simulink model "cic"  (Simulink 6.3)
settings: Solver=FixedStepDiscrete  SolverMode=SingleTasking  StartTime=0.0  StopTime=1000  RelTol=1e-3
InitFcn:
  | %% DSPBuilder Start
  | alt_dspbuilder_update_model(bdroot)
  | %% DSPBuilder End
libraries: allblocks_alteradspbuilder2 x32
settings Model: Creator=mjervis  LastModifiedBy=LKONG
settings DataIOCC: SignalLoggingName=sigsOut
settings OptimizationCC: BooleanDataType=off  InlineInvariantSignals=on
settings DebuggingCC: SolverPrmCheckMsg=none
settings HardwareCC: TargetUnknown=on

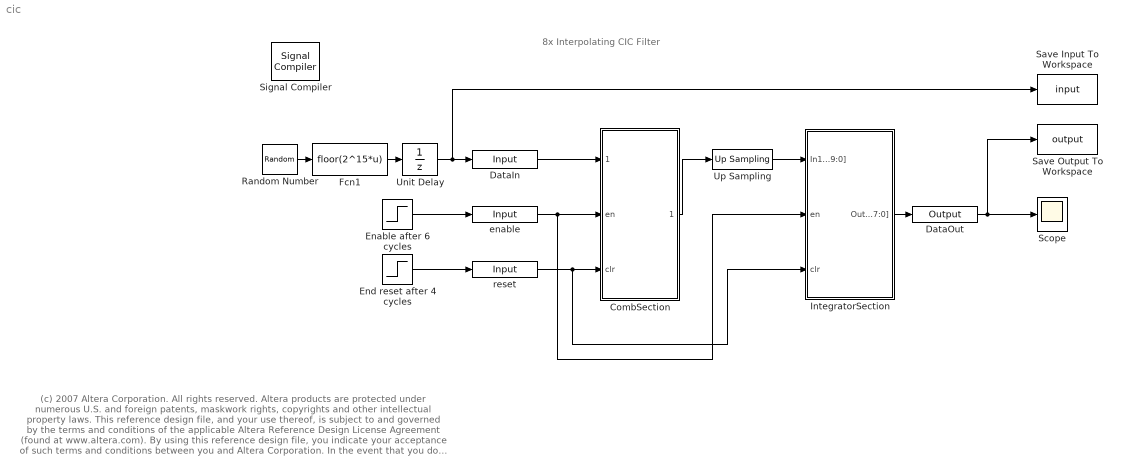
== system cic ==
  note: 8x Interpolating CIC Filter
  note: (c) 2007 Altera Corporation. All rights reserved.  Altera products are protected under numerous U.S. and foreign patents, maskwork rights, copyrights and other intellectual property laws.
      | This reference design file, and your use thereof, is subject to and governed by the terms and conditions of the applicable Altera Reference Design License Agreement (found at www.altera.com).
      | By using this reference design file, you indicate your acceptance of such terms and conditions between you and Altera Corporation.
      | In the event that you do not agree with such terms and conditions, you may not use the reference design file and please promptly destroy any copies you have made.
      | This reference design file being provided on an "as-is" basis and as an accommodation and therefore all warranties, representations or guarantees of any kind (whether express, implied or statutory)
      | including, without limitation, warranties of merchantability, non-infringement, or fitness for a particular purpose, are specifically disclaimed.
      | By making this reference design file available, Altera expressly does not recommend, suggest or require that this reference design file be used in combination with any other product not provided by Altera
  CombSection : Subsystem  AncestorBlock=ALTELINK/AltLab/HDL SubSystem
      mask Type: SubSystem AlteraBlockSet
  DataIn : allblocks_alteradspbuilder2/Input  iofile=D:\wsTrunk\workspace\Documentation\DesignExamples\Demos\Filters\CicFilter\Cic\tb_cic\cic_DataIn.salt  BusType=Signed Integer  bwl=16  bwr=0  SpecifyClock=off  PORTTYPE=Input
  DataOut : allblocks_alteradspbuilder2/Output  iofile=D:\wsTrunk\workspace\Documentation\DesignExamples\Demos\Filters\CicFilter\Cic\tb_cic\cic_DataOut.capture  BusType=Signed Integer  bwl=28  bwr=0  PORTTYPE=Output
  Enable after 6 cycles : Step  Time=6  SampleTime=1
  End reset after 4 cycles : Step  Time=4  Before=1  After=0  SampleTime=1
  Fcn1 : Fcn  Expr=floor(2^15*u)
  IntegratorSection : Subsystem  AncestorBlock=ALTELINK/AltLab/HDL SubSystem
      mask Type: SubSystem AlteraBlockSet
  Random Number : RandomNumber  Variance=8  SampleTime=8
  Save Input To Workspace : ToWorkspace  VariableName=input  SampleTime=-1  SaveFormat=Array
  Save Output To Workspace : ToWorkspace  VariableName=output  SampleTime=-1  SaveFormat=Array
  Scope : Scope
      settings: TimeRange=1000  YMin=-150000000  YMax=150000000  SaveName=ScopeData2
  Signal Compiler : allblocks_alteradspbuilder2/Signal Compiler  DeviceFamily=Stratix IV  DeviceName=AUTO  EnableSignalTap=off  SignalTapDepth=128  UseBoardBlock=off  StpUseDefaultClock=on  StpClock=Clock
  Unit Delay : UnitDelay  SampleTime=8
  Up Sampling : allblocks_alteradspbuilder2/Up Sampling  rate=8
  enable : allblocks_alteradspbuilder2/Input  iofile=D:\wsTrunk\workspace\Documentation\DesignExamples\Demos\Filters\CicFilter\Cic\tb_cic\cic_enable.salt  BusType=Single Bit  bwl=1  bwr=0  SpecifyClock=off  PORTTYPE=Input
  reset : allblocks_alteradspbuilder2/Input  iofile=D:\wsTrunk\workspace\Documentation\DesignExamples\Demos\Filters\CicFilter\Cic\tb_cic\cic_reset.salt  BusType=Single Bit  bwl=1  bwr=0  SpecifyClock=off  PORTTYPE=Input
  wires:
  Up Sampling/1 -> IntegratorSection/1(In1[19:0])
  IntegratorSection/1(Out1[27:0]) -> DataOut/1
  DataOut/1 -> Scope/1, Save Output To Workspace/1
  Random Number/1 -> Fcn1/1
  Unit Delay/1 -> DataIn/1, Save Input To Workspace/1
  Fcn1/1 -> Unit Delay/1
  CombSection/1(Out1[20:0]) -> Up Sampling/1
  Enable after 6 cycles/1 -> enable/1
  End reset after 4 cycles/1 -> reset/1
  DataIn/1 -> CombSection/1(In1[16:0])
  enable/1 -> CombSection/2(en), IntegratorSection/2(en)
  reset/1 -> IntegratorSection/3(clr), CombSection/3(clr)

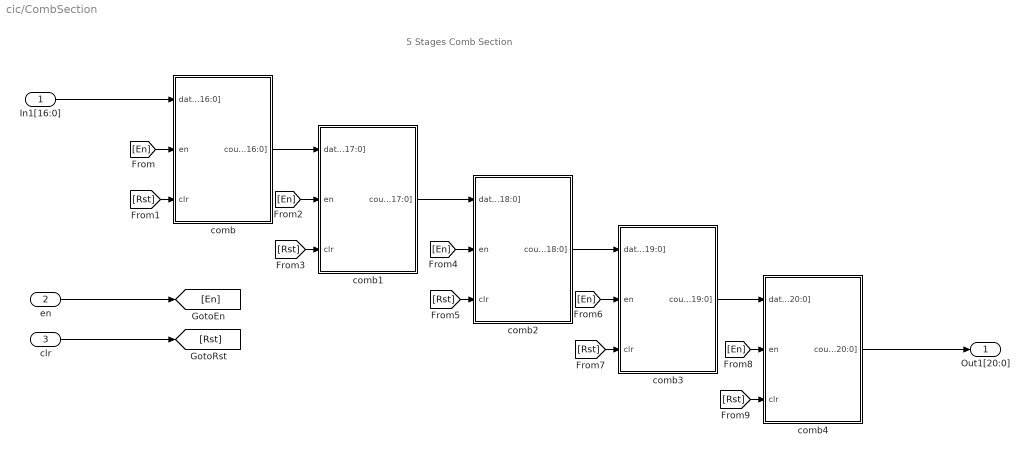
== system cic/CombSection ==
  note: 5 Stages Comb Section
  In1[16:0] : Inport
  en : Inport  Port=2
  clr : Inport  Port=3
  comb : Subsystem  AncestorBlock=ALTELINK/AltLab/HDL SubSystem
      mask Type: SubSystem AlteraBlockSet
  comb1 : Subsystem  AncestorBlock=ALTELINK/AltLab/HDL SubSystem
      mask Type: SubSystem AlteraBlockSet
  comb2 : Subsystem  AncestorBlock=ALTELINK/AltLab/HDL SubSystem
      mask Type: SubSystem AlteraBlockSet
  comb3 : Subsystem  AncestorBlock=ALTELINK/AltLab/HDL SubSystem
      mask Type: SubSystem AlteraBlockSet
  comb4 : Subsystem  AncestorBlock=ALTELINK/AltLab/HDL SubSystem
      mask Type: SubSystem AlteraBlockSet
  Out1[20:0] : Outport
  wires:
  In1[16:0]/1 -> comb/1(data[16:0])
  comb/1(cout[16:0]) -> comb1/1(data[17:0])
  comb1/1(cout[17:0]) -> comb2/1(data[18:0])
  comb2/1(cout[18:0]) -> comb3/1(data[19:0])
  comb3/1(cout[19:0]) -> comb4/1(data[20:0])
  comb4/1(cout[20:0]) -> Out1[20:0]/1
  en/1 -> [En]
  clr/1 -> [Rst]
  [En] -> comb/2(en)
  [Rst] -> comb/3(clr)
  [En] -> comb4/2(en)
  [Rst] -> comb4/3(clr)
  [En] -> comb3/2(en)
  [Rst] -> comb3/3(clr)
  [En] -> comb2/2(en)
  [Rst] -> comb2/3(clr)
  [En] -> comb1/2(en)
  [Rst] -> comb1/3(clr)

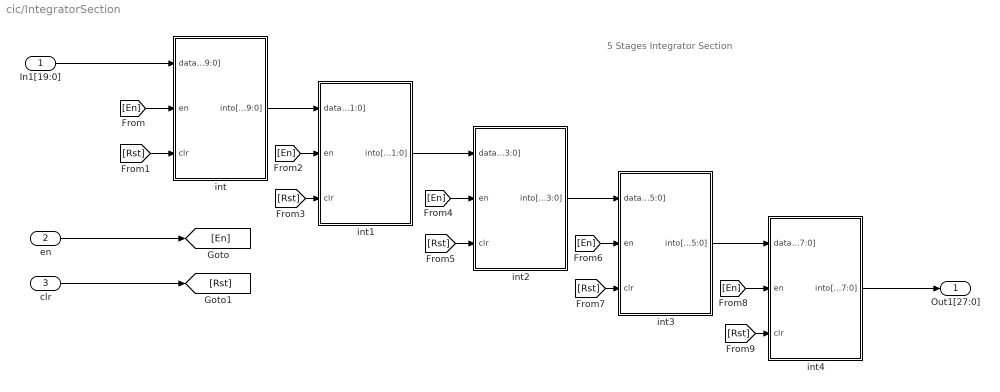
== system cic/IntegratorSection ==
  note: 5 Stages Integrator Section
  In1[19:0] : Inport
  en : Inport  Port=2
  clr : Inport  Port=3
  int : Subsystem  AncestorBlock=ALTELINK/AltLab/HDL SubSystem
      mask Type: SubSystem AlteraBlockSet
  int1 : Subsystem  AncestorBlock=ALTELINK/AltLab/HDL SubSystem
      mask Type: SubSystem AlteraBlockSet
  int2 : Subsystem  AncestorBlock=ALTELINK/AltLab/HDL SubSystem
      mask Type: SubSystem AlteraBlockSet
  int3 : Subsystem  AncestorBlock=ALTELINK/AltLab/HDL SubSystem
      mask Type: SubSystem AlteraBlockSet
  int4 : Subsystem  AncestorBlock=ALTELINK/AltLab/HDL SubSystem
      mask Type: SubSystem AlteraBlockSet
  Out1[27:0] : Outport
  wires:
  In1[19:0]/1 -> int/1(data[19:0])
  int/1(into[19:0]) -> int1/1(data[21:0])
  int1/1(into[21:0]) -> int2/1(data[23:0])
  int2/1(into[23:0]) -> int3/1(data[25:0])
  int3/1(into[25:0]) -> int4/1(data[27:0])
  en/1 -> [En]
  clr/1 -> [Rst]
  int4/1(into[27:0]) -> Out1[27:0]/1
  [En] -> int/2(en)
  [Rst] -> int/3(clr)
  [En] -> int4/2(en)
  [Rst] -> int4/3(clr)
  [En] -> int3/2(en)
  [Rst] -> int3/3(clr)
  [En] -> int2/2(en)
  [Rst] -> int2/3(clr)
  [En] -> int1/2(en)
  [Rst] -> int1/3(clr)

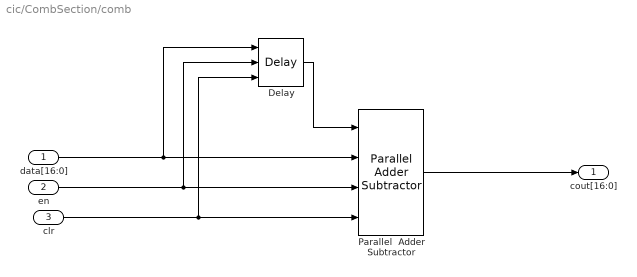
== system cic/CombSection/comb ==
  data[16:0] : Inport
  en : Inport  Port=2
  clr : Inport  Port=3
  Delay : allblocks_alteradspbuilder2/Delay  pipeline=1  ClockPhase=10000000  use_ena=on  use_sclr=on  use_init=off  reset_value=1
  Parallel  Adder Subtractor : allblocks_alteradspbuilder2/Parallel Adder Subtractor  number_of_inputs=2  direction=-  use_pipeline=on  phase_selection=10000000  use_ena=on  use_aclr=on
  cout[16:0] : Outport
  wires:
  Delay/1 -> Parallel  Adder Subtractor/1
  Parallel  Adder Subtractor/1 -> cout[16:0]/1
  en/1 -> Parallel  Adder Subtractor/3, Delay/2
  clr/1 -> Parallel  Adder Subtractor/4, Delay/3
  data[16:0]/1 -> Parallel  Adder Subtractor/2, Delay/1

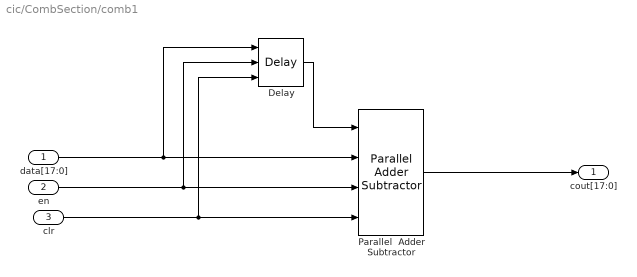
== system cic/CombSection/comb1 ==
  data[17:0] : Inport
  en : Inport  Port=2
  clr : Inport  Port=3
  Delay : allblocks_alteradspbuilder2/Delay  pipeline=1  ClockPhase=10000000  use_ena=on  use_sclr=on  use_init=off  reset_value=1
  Parallel  Adder Subtractor : allblocks_alteradspbuilder2/Parallel Adder Subtractor  number_of_inputs=2  direction=-  use_pipeline=on  phase_selection=10000000  use_ena=on  use_aclr=on
  cout[17:0] : Outport
  wires:
  Delay/1 -> Parallel  Adder Subtractor/1
  Parallel  Adder Subtractor/1 -> cout[17:0]/1
  en/1 -> Parallel  Adder Subtractor/3, Delay/2
  clr/1 -> Parallel  Adder Subtractor/4, Delay/3
  data[17:0]/1 -> Parallel  Adder Subtractor/2, Delay/1

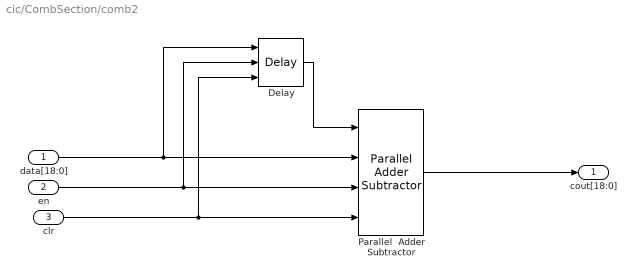
== system cic/CombSection/comb2 ==
  data[18:0] : Inport
  en : Inport  Port=2
  clr : Inport  Port=3
  Delay : allblocks_alteradspbuilder2/Delay  pipeline=1  ClockPhase=10000000  use_ena=on  use_sclr=on  use_init=off  reset_value=1
  Parallel  Adder Subtractor : allblocks_alteradspbuilder2/Parallel Adder Subtractor  number_of_inputs=2  direction=-  use_pipeline=on  phase_selection=10000000  use_ena=on  use_aclr=on
  cout[18:0] : Outport
  wires:
  data[18:0]/1 -> Delay/1, Parallel  Adder Subtractor/2
  clr/1 -> Delay/3, Parallel  Adder Subtractor/4
  en/1 -> Delay/2, Parallel  Adder Subtractor/3
  Parallel  Adder Subtractor/1 -> cout[18:0]/1
  Delay/1 -> Parallel  Adder Subtractor/1

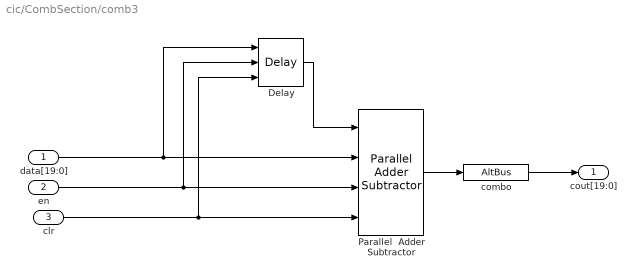
== system cic/CombSection/comb3 ==
  data[19:0] : Inport
  en : Inport  Port=2
  clr : Inport  Port=3
  Delay : allblocks_alteradspbuilder2/Delay  pipeline=1  ClockPhase=10000000  use_ena=on  use_sclr=on  use_init=off  reset_value=1
  Parallel  Adder Subtractor : allblocks_alteradspbuilder2/Parallel Adder Subtractor  number_of_inputs=2  direction=-  use_pipeline=on  phase_selection=10000000  use_ena=on  use_aclr=on
  combo : allblocks_alteradspbuilder2/AltBus  BusType=Signed Integer  bwl=20  bwr=0  saturate=off
  cout[19:0] : Outport
  wires:
  Delay/1 -> Parallel  Adder Subtractor/1
  Parallel  Adder Subtractor/1 -> combo/1
  en/1 -> Parallel  Adder Subtractor/3, Delay/2
  clr/1 -> Parallel  Adder Subtractor/4, Delay/3
  data[19:0]/1 -> Parallel  Adder Subtractor/2, Delay/1
  combo/1 -> cout[19:0]/1

== system cic/CombSection/comb4 ==
  data[20:0] : Inport
  en : Inport  Port=2
  clr : Inport  Port=3
  Delay : allblocks_alteradspbuilder2/Delay  pipeline=1  ClockPhase=10000000  use_ena=on  use_sclr=on  use_init=off  reset_value=1
  Parallel  Adder Subtractor : allblocks_alteradspbuilder2/Parallel Adder Subtractor  number_of_inputs=2  direction=-  use_pipeline=on  phase_selection=10000000  use_ena=on  use_aclr=on
  cout[20:0] : Outport
  wires:
  data[20:0]/1 -> Delay/1, Parallel  Adder Subtractor/2
  clr/1 -> Delay/3, Parallel  Adder Subtractor/4
  en/1 -> Delay/2, Parallel  Adder Subtractor/3
  Parallel  Adder Subtractor/1 -> cout[20:0]/1
  Delay/1 -> Parallel  Adder Subtractor/1

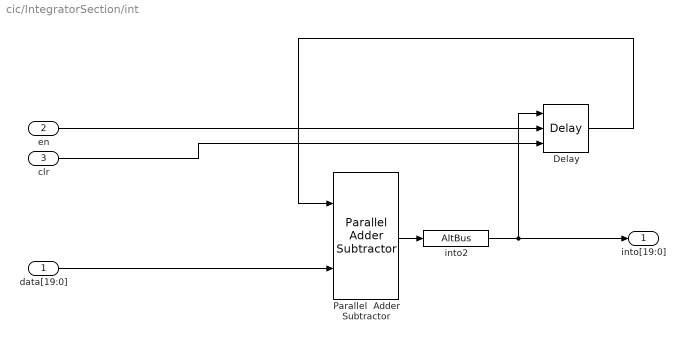
== system cic/IntegratorSection/int ==
  data[19:0] : Inport
  en : Inport  Port=2
  clr : Inport  Port=3
  Delay : allblocks_alteradspbuilder2/Delay  pipeline=1  ClockPhase=1  use_ena=on  use_sclr=on  use_init=off  reset_value=1
  Parallel  Adder Subtractor : allblocks_alteradspbuilder2/Parallel Adder Subtractor  number_of_inputs=2  direction=+  use_pipeline=off  phase_selection=1  use_ena=off  use_aclr=off
  into2 : allblocks_alteradspbuilder2/AltBus  BusType=Signed Integer  bwl=20  bwr=0  saturate=off
  into[19:0] : Outport
  wires:
  data[19:0]/1 -> Parallel  Adder Subtractor/2
  Parallel  Adder Subtractor/1 -> into2/1
  en/1 -> Delay/2
  clr/1 -> Delay/3
  Delay/1 -> Parallel  Adder Subtractor/1
  into2/1 -> Delay/1, into[19:0]/1

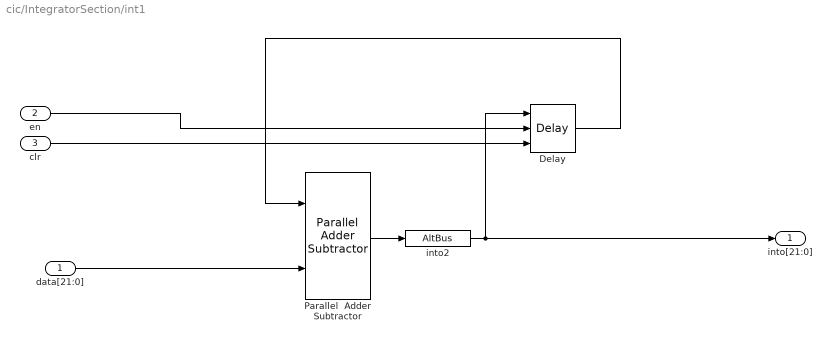
== system cic/IntegratorSection/int1 ==
  data[21:0] : Inport
  en : Inport  Port=2
  clr : Inport  Port=3
  Delay : allblocks_alteradspbuilder2/Delay  pipeline=1  ClockPhase=1  use_ena=on  use_sclr=on  use_init=off  reset_value=1
  Parallel  Adder Subtractor : allblocks_alteradspbuilder2/Parallel Adder Subtractor  number_of_inputs=2  direction=+  use_pipeline=off  phase_selection=1  use_ena=on  use_aclr=on
  into2 : allblocks_alteradspbuilder2/AltBus  BusType=Signed Integer  bwl=22  bwr=0  saturate=off
  into[21:0] : Outport
  wires:
  Delay/1 -> Parallel  Adder Subtractor/1
  clr/1 -> Delay/3
  en/1 -> Delay/2
  Parallel  Adder Subtractor/1 -> into2/1
  data[21:0]/1 -> Parallel  Adder Subtractor/2
  into2/1 -> Delay/1, into[21:0]/1

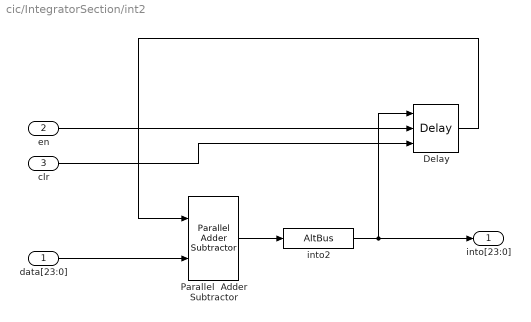
== system cic/IntegratorSection/int2 ==
  data[23:0] : Inport
  en : Inport  Port=2
  clr : Inport  Port=3
  Delay : allblocks_alteradspbuilder2/Delay  pipeline=1  ClockPhase=1  use_ena=on  use_sclr=on  use_init=off  reset_value=1
  Parallel  Adder Subtractor : allblocks_alteradspbuilder2/Parallel Adder Subtractor  number_of_inputs=2  direction=+  use_pipeline=off  phase_selection=1  use_ena=on  use_aclr=on
  into2 : allblocks_alteradspbuilder2/AltBus  BusType=Signed Integer  bwl=24  bwr=0  saturate=off
  into[23:0] : Outport
  wires:
  data[23:0]/1 -> Parallel  Adder Subtractor/2
  Parallel  Adder Subtractor/1 -> into2/1
  clr/1 -> Delay/3
  Delay/1 -> Parallel  Adder Subtractor/1
  into2/1 -> Delay/1, into[23:0]/1
  en/1 -> Delay/2

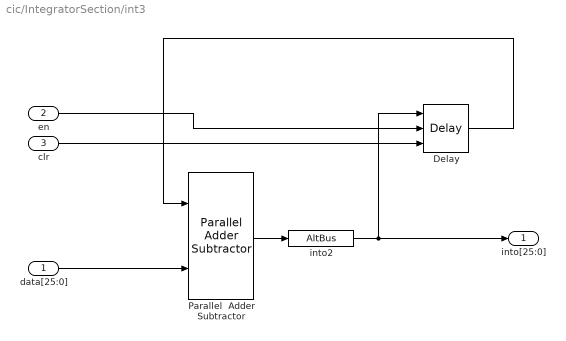
== system cic/IntegratorSection/int3 ==
  data[25:0] : Inport
  en : Inport  Port=2
  clr : Inport  Port=3
  Delay : allblocks_alteradspbuilder2/Delay  pipeline=1  ClockPhase=1  use_ena=on  use_sclr=on  use_init=off  reset_value=1
  Parallel  Adder Subtractor : allblocks_alteradspbuilder2/Parallel Adder Subtractor  number_of_inputs=2  direction=+  use_pipeline=off  phase_selection=1  use_ena=on  use_aclr=on
  into2 : allblocks_alteradspbuilder2/AltBus  BusType=Signed Integer  bwl=26  bwr=0  saturate=off
  into[25:0] : Outport
  wires:
  Delay/1 -> Parallel  Adder Subtractor/1
  clr/1 -> Delay/3
  en/1 -> Delay/2
  Parallel  Adder Subtractor/1 -> into2/1
  data[25:0]/1 -> Parallel  Adder Subtractor/2
  into2/1 -> Delay/1, into[25:0]/1

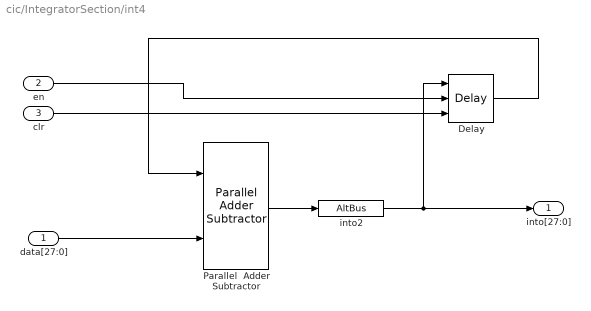
== system cic/IntegratorSection/int4 ==
  data[27:0] : Inport
  en : Inport  Port=2
  clr : Inport  Port=3
  Delay : allblocks_alteradspbuilder2/Delay  pipeline=1  ClockPhase=1  use_ena=on  use_sclr=on  use_init=off  reset_value=1
  Parallel  Adder Subtractor : allblocks_alteradspbuilder2/Parallel Adder Subtractor  number_of_inputs=2  direction=+  use_pipeline=off  phase_selection=1  use_ena=on  use_aclr=on
  into2 : allblocks_alteradspbuilder2/AltBus  BusType=Signed Integer  bwl=28  bwr=0  saturate=off
  into[27:0] : Outport
  wires:
  data[27:0]/1 -> Parallel  Adder Subtractor/2
  Parallel  Adder Subtractor/1 -> into2/1
  en/1 -> Delay/2
  clr/1 -> Delay/3
  Delay/1 -> Parallel  Adder Subtractor/1
  into2/1 -> Delay/1, into[27:0]/1
